simulink model "pll_stability_9bus"  (R2025b)
settings: Solver=ode23t  StartTime=0.0  StopTime=0.6  FixedStep=Ts  RelTol=1e-3  EnableMultiTasking=on
InitFcn:
  | proj_root = fileparts(get_param(bdroot, 'FileName'));
  | run(fullfile(proj_root, 'params.m'))
StopFcn:
  | run(fullfile(fileparts(get_param(bdroot, 'FileName')), 'scripts', 'export_sim_data.m'))
values from neighbouring files (symbols this model uses):
  C1 = 4.247098756978487e-05    (= 4.24709875698e-05)    [GridTiedInverterOptimalIData.m]    (also in params.m)
  den_notch_d = [1.0, -1.9198159829792367, 0.9417686752314415]    [params.m]
  Ki = 7075.557375636462 /4    (= 1768.88934391)    [GridTiedInverterOptimalIData.m]    (also in params.m)
  ki_pll = ki_pll * 0.2    (= 21164)    [params.m]
  Kp = 29.481489065151926 /4    (= 7.37037226629)    [GridTiedInverterOptimalIData.m]    (also in params.m)
  kp_pll = kp_pll * 0.2    (= 92)    [params.m]
  L1 = 0.03042088602562317    (= 0.0304208860256)    [GridTiedInverterOptimalIData.m]    (also in params.m)
  L2 = 0.0002889984172434201    (= 0.000288998417243)    [GridTiedInverterOptimalIData.m]    (also in params.m)
  num_notch_d = [0.9723401207349347, -1.9198159829792367, 0.9694285544965067]    [params.m]
  qsi = 0.707    [GridTiedInverterOptimalIData.m]    (also in params.m)
  Rd1 = 0.5734201923227409    (= 0.573420192323)    [GridTiedInverterOptimalIData.m]    (also in params.m)
  Rd2 = 0.0054474918270660385    (= 0.00544749182707)    [GridTiedInverterOptimalIData.m]    (also in params.m)
  Rd3 = 3.1228169353331086    (= 3.12281693533)    [GridTiedInverterOptimalIData.m]    (also in params.m)
  Ts = 5e-6    (= 5e-06)    [GridTiedInverterOptimalIData.m]    (also in params.m)
  Tsc = 2e-4    (= 0.0002)    [GridTiedInverterOptimalIData.m]    (also in params.m)
  Vcc = 90909.09090909091*1.5    (= 136363.636364)    [GridTiedInverterOptimalIData.m]    (also in params.m)
  wres = 9068.99682117109    (= 9068.99682117)    [GridTiedInverterOptimalIData.m]    (also in params.m)
libraries: nesl_utility x80, ee_lib x71, fl_lib x28, eeGeneralControl x9, eeTransforms x4, eeSmAC1C x3, eeSmPSS1A x3, simulink x3, eeSinusoidalMeasurement x1
(part 3 of 3)

== system pll_stability_9bus/Gen3@Bus3 PV 1.025 pu 85 MW/Governor and Prime Mover ==
  "Governor and Prime Mover " : Subsystem  mask(Governor and Prime Mover){droop_percentage=5, Tg=0.15, Tch=0.3, pu_torque0=0.668315, Ts=Ts}
      mask prompts: droop_percentage "Percentage droop, (%)"; Tg "Time constant of governor, Tg (s)"; Tch "Time constant of main inlet volumes and steam chest, Tch (s)"; pu_torque0 "Initial torque, (pu)"; Ts "Sample time"
      mask help:
      | Implements a synchronous machine governor and prime mover. The prime mover is a non-reheat steam turbine.
      |
      | The input to the block is a per-unit synchronous machine measurement vector.
      |
      | R and C are mechanical rotational ports.
  Mechanical Power : ee_lib/Electromechanical/Mechanical/Machine Mechanical Power  power_sign=-1  SRated=128 MW  FRated=60 Hz  nPolePairs=1  inputUnit=ee.enum.unit.pu  torque_factor=2  inertia_option=2  J=27548 kg*m^2  H=301/128 W*s/(A*V)  damper_option=2  D=39.0509 N*m*s/rad  pu_D=0  initialization_option=2  fMechanical0=60 Hz  fElectrical0=60 Hz
      settings: InternalSimscapePortConfiguration="{\"Bottom\":[],\"Left\":[{\"id\":\"Pm_pu\",\"label\":\"pu\",\"type\":\"input\"}],\"Right\":[{\"id\":\"R\",\"label\":\"R\",\"type\":\"foundation.mechanical.rotational.rotational\"},{\"id\":\"C\",\"label\":\"C\",\"type\":\"foundation.mechanical.rotational.rotational\"}],\"Top\":[]}"
  PS-Simulink Converter : nesl_utility/PS-Simulink Converter  PhysicalDomain=network_engine_domain  SubClassName=ps_output  LeftPortType=input  RightPortType=output  PseudoPeriodic=off  Frequencies=[]  VectorFormat=1-D array  Unit=1  AffineConversion=off
  Pref : Constant  Value=85/128
  Rotor velocity measurement : ee_lib/Electromechanical/Synchronous/Synchronous Machine Measurement  output_idx=4
      settings: InternalSimscapePortConfiguration="{\"Bottom\":[],\"Left\":[{\"id\":\"pu_input\",\"label\":\"pu\",\"type\":\"input\"}],\"Right\":[{\"id\":\"pu_output\",\"label\":\"o\",\"type\":\"output\"}],\"Top\":[]}"
  Simulink-PS Converter : nesl_utility/Simulink-PS Converter  PhysicalDomain=network_engine_domain  SubClassName=ps_input  LeftPortType=input  RightPortType=output  PseudoPeriodic=off  Frequencies=[]  NoiseDistribution=none  NoiseParameters=[]  Unit=1  AffineConversion=off  FilteringAndDerivatives=provide  SimscapeFilterOrder=1  InputFilterTimeConstant=0.001  UdotUserProvided=0
  Unit Delay : UnitDelay  InitialCondition=1  SampleTime=Ts  HasFrameUpgradeWarning=on
  wref : Constant
  R : PMIOPort  Side=Right
  C : PMIOPort  Port=2  Side=Right
  pu : PMIOPort  Port=3  Side=Left
  wires:
  PS-Simulink Converter/1 -> Unit Delay/1
  Unit Delay/1 -> "Governor and Prime Mover "/3(w)
  Pref/1 -> "Governor and Prime Mover "/2(Pref)
  "Governor and Prime Mover "/1(Tm) -> Simulink-PS Converter/1
  wref/1 -> "Governor and Prime Mover "/1(wref)
  connections:
  PS-Simulink Converter/LConn1 -- Rotor velocity measurement/RConn1
  Mechanical Power/RConn1 -- R/RConn1
  pu/RConn1 -- Rotor velocity measurement/LConn1
  Mechanical Power/RConn2 -- C/RConn1
  Mechanical Power/LConn1 -- Simulink-PS Converter/RConn1

== system pll_stability_9bus/UFV Model/Gate driver ==
  S : Inport
  Data Type Conversion : DataTypeConversion  OutDataTypeStr=double  SaturateOnIntegerOverflow=off  RndMeth=Floor
  Demux : Demux  Outputs=6
  Scope : Scope
      settings: ActiveDisplayYMinimum=-0.036991199119911888  ActiveDisplayYMaximum=1.0342409240924093  DataLoggingVariableName=ScopeData3
  Simulink-PS Converter{,1..5} (6 alike) : nesl_utility/Simulink-PS Converter  PhysicalDomain=network_engine_domain  SubClassName=ps_input  LeftPortType=input  RightPortType=output  PseudoPeriodic=off  Frequencies=[]  NoiseDistribution=none  NoiseParameters=[]  Unit=1  AffineConversion=off  FilteringAndDerivatives=provide  SimscapeFilterOrder=1  InputFilterTimeConstant=0.001  UdotUserProvided=0
  Six-Pulse Gate Multiplexer : ee_lib/Semiconductors & Converters/Converters/Six-Pulse Gate Multiplexer  port_option=ee.enum.controlport.ps
  G : PMIOPort  Side=Right
  wires:
  Demux/5 -> Simulink-PS Converter4/1
  Demux/3 -> Simulink-PS Converter2/1
  Data Type Conversion/1 -> Demux/1
  Demux/4 -> Simulink-PS Converter3/1
  Demux/6 -> Simulink-PS Converter5/1
  Demux/2 -> Simulink-PS Converter1/1
  Demux/1 -> Scope/1, Simulink-PS Converter/1
  S/1 -> Data Type Conversion/1
  connections:
  Simulink-PS Converter4/RConn1 -- Six-Pulse Gate Multiplexer/LConn5
  Simulink-PS Converter2/RConn1 -- Six-Pulse Gate Multiplexer/LConn3
  Simulink-PS Converter/RConn1 -- Six-Pulse Gate Multiplexer/LConn1
  Simulink-PS Converter5/RConn1 -- Six-Pulse Gate Multiplexer/LConn6
  Simulink-PS Converter1/RConn1 -- Six-Pulse Gate Multiplexer/LConn2
  Simulink-PS Converter3/RConn1 -- Six-Pulse Gate Multiplexer/LConn4
  Six-Pulse Gate Multiplexer/RConn1 -- G/RConn1

== system pll_stability_9bus/UFV Model/Measurement inverter ==
  Current and Voltage Sensor (Three-Phase) : ee_lib/Sensors & Transducers/Current and Voltage Sensor (Three-Phase)  vMeasurementType=2  outputUnit=1  SRated=100e6 V*A  VRated=18e3 V  I_specify=off  I_priority=None  I=[ 0 0 0 ] A  I_nominal_specify=off  I_nominal_value=1  I_nominal_unit=A  V_specify=off  V_priority=None  V=[ 0 0 0 ] V  V_nominal_specify=off  V_nominal_value=1  V_nominal_unit=V
      settings: InternalSimscapePortConfiguration="{\"Bottom\":[],\"Left\":[{\"id\":\"a1\",\"label\":\"a1\",\"type\":\"foundation.electrical.electrical\"},{\"id\":\"b1\",\"label\":\"b1\",\"type\":\"foundation.electrical.electrical\"},{\"id\":\"c1\",\"label\":\"c1\",\"type\":\"foundation.electrical.electrical\"}],\"Right\":[{\"id\":\"V_output\",\"label\":\"V\",\"type\":\"output\"},{\"id\":\"I_output\",\"label\":\"I\",\"type\":\"output\"},{\"id\":\"a2\",\"label\":\"a2\",\"type\":\"foundation.electrical.electrical\"},{\"id\":\"b2\",\"label\":\"b2\",\"type\":\"foundation.electrical.electrical\"},{\"id\":\"c2\",\"label\":\"c2\",\"type\":\"foundation.electrical.electrical\"}],\"Top\":[]}"
  PS-Simulink Converter : nesl_utility/PS-Simulink Converter  PhysicalDomain=network_engine_domain  SubClassName=ps_output  LeftPortType=input  RightPortType=output  PseudoPeriodic=off  Frequencies=[]  VectorFormat=1-D array  Unit=V  AffineConversion=off
  PS-Simulink Converter2 : nesl_utility/PS-Simulink Converter  PhysicalDomain=network_engine_domain  SubClassName=ps_output  LeftPortType=input  RightPortType=output  PseudoPeriodic=off  Frequencies=[]  VectorFormat=1-D array  Unit=1  AffineConversion=off
  PS-Simulink Converter3 : nesl_utility/PS-Simulink Converter  PhysicalDomain=network_engine_domain  SubClassName=ps_output  LeftPortType=input  RightPortType=output  PseudoPeriodic=off  Frequencies=[]  VectorFormat=1-D array  Unit=1  AffineConversion=off
  Voltage Sensor : fl_lib/Electrical/Electrical Sensors/Voltage Sensor
  a1 : PMIOPort  Side=Left
  b1 : PMIOPort  Port=2  Side=Left
  a2 : PMIOPort  Port=3  Side=Right
  b2 : PMIOPort  Port=4  Side=Right
  c1 : PMIOPort  Port=5  Side=Left
  c2 : PMIOPort  Port=6  Side=Right
  tag scope: Iabc_inverter=global, Vab_inverter=global, Vabc_inverter=global
  wires:
  PS-Simulink Converter3/1 -> [Iabc_inverter]
  PS-Simulink Converter/1 -> [Vab_inverter]
  PS-Simulink Converter2/1 -> [Vabc_inverter]
  connections:
  b2/RConn1 -- Voltage Sensor/RConn2 -- Current and Voltage Sensor (Three-Phase)/RConn4
  a2/RConn1 -- Voltage Sensor/LConn1 -- Current and Voltage Sensor (Three-Phase)/RConn3
  Current and Voltage Sensor (Three-Phase)/RConn5 -- c2/RConn1
  Current and Voltage Sensor (Three-Phase)/LConn2 -- b1/RConn1
  Current and Voltage Sensor (Three-Phase)/LConn3 -- c1/RConn1
  Current and Voltage Sensor (Three-Phase)/LConn1 -- a1/RConn1
  PS-Simulink Converter2/LConn1 -- Current and Voltage Sensor (Three-Phase)/RConn1
  Current and Voltage Sensor (Three-Phase)/RConn2 -- PS-Simulink Converter3/LConn1
  PS-Simulink Converter/LConn1 -- Voltage Sensor/RConn1

== system pll_stability_9bus/UFV Model/Measurement inverter1 ==
  Current and Voltage Sensor (Three-Phase) : ee_lib/Sensors & Transducers/Current and Voltage Sensor (Three-Phase)  vMeasurementType=2  outputUnit=ee.enum.unit.si  SRated=100e6 V*A  VRated=20e3 V  I_specify=off  I_priority=None  I=[ 0 0 0 ] A  I_nominal_specify=off  I_nominal_value=1  I_nominal_unit=A  V_specify=off  V_priority=None  V=[ 0 0 0 ] V  V_nominal_specify=off  V_nominal_value=1  V_nominal_unit=V
      settings: InternalSimscapePortConfiguration="{\"Bottom\":[],\"Left\":[{\"id\":\"a1\",\"label\":\"a1\",\"type\":\"foundation.electrical.electrical\"},{\"id\":\"b1\",\"label\":\"b1\",\"type\":\"foundation.electrical.electrical\"},{\"id\":\"c1\",\"label\":\"c1\",\"type\":\"foundation.electrical.electrical\"}],\"Right\":[{\"id\":\"V_output\",\"label\":\"V\",\"type\":\"output\"},{\"id\":\"I_output\",\"label\":\"I\",\"type\":\"output\"},{\"id\":\"a2\",\"label\":\"a2\",\"type\":\"foundation.electrical.electrical\"},{\"id\":\"b2\",\"label\":\"b2\",\"type\":\"foundation.electrical.electrical\"},{\"id\":\"c2\",\"label\":\"c2\",\"type\":\"foundation.electrical.electrical\"}],\"Top\":[]}"
  PS-Simulink Converter : nesl_utility/PS-Simulink Converter  PhysicalDomain=network_engine_domain  SubClassName=ps_output  LeftPortType=input  RightPortType=output  PseudoPeriodic=off  Frequencies=[]  VectorFormat=1-D array  Unit=V  AffineConversion=off
  PS-Simulink Converter2 : nesl_utility/PS-Simulink Converter  PhysicalDomain=network_engine_domain  SubClassName=ps_output  LeftPortType=input  RightPortType=output  PseudoPeriodic=off  Frequencies=[]  VectorFormat=1-D array  Unit=1  AffineConversion=off
  PS-Simulink Converter3 : nesl_utility/PS-Simulink Converter  PhysicalDomain=network_engine_domain  SubClassName=ps_output  LeftPortType=input  RightPortType=output  PseudoPeriodic=off  Frequencies=[]  VectorFormat=1-D array  Unit=1  AffineConversion=off
  Voltage Sensor : fl_lib/Electrical/Electrical Sensors/Voltage Sensor
  a1 : PMIOPort  Side=Left
  b1 : PMIOPort  Port=2  Side=Left
  a2 : PMIOPort  Port=3  Side=Right
  b2 : PMIOPort  Port=4  Side=Right
  c1 : PMIOPort  Port=5  Side=Left
  c2 : PMIOPort  Port=6  Side=Right
  tag scope: Iabc=global, Vab=global, Vabc=global
  wires:
  PS-Simulink Converter2/1 -> [Vabc]
  PS-Simulink Converter3/1 -> [Iabc]
  PS-Simulink Converter/1 -> [Vab]
  connections:
  b2/RConn1 -- Voltage Sensor/RConn2 -- Current and Voltage Sensor (Three-Phase)/RConn4
  a2/RConn1 -- Voltage Sensor/LConn1 -- Current and Voltage Sensor (Three-Phase)/RConn3
  Current and Voltage Sensor (Three-Phase)/RConn5 -- c2/RConn1
  Current and Voltage Sensor (Three-Phase)/LConn2 -- b1/RConn1
  Current and Voltage Sensor (Three-Phase)/LConn3 -- c1/RConn1
  Current and Voltage Sensor (Three-Phase)/LConn1 -- a1/RConn1
  PS-Simulink Converter2/LConn1 -- Current and Voltage Sensor (Three-Phase)/RConn1
  Current and Voltage Sensor (Three-Phase)/RConn2 -- PS-Simulink Converter3/LConn1
  PS-Simulink Converter/LConn1 -- Voltage Sensor/RConn1

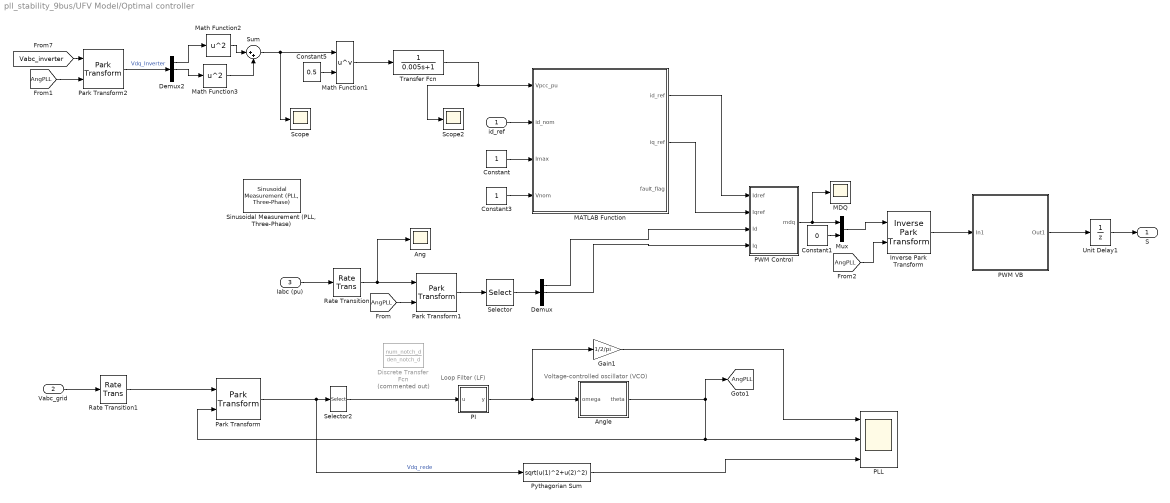
== system pll_stability_9bus/UFV Model/Optimal controller ==
  note: Loop Filter (LF)
  note: Voltage-controlled oscillator (VCO)
  id_ref : Inport
  Vabc_grid : Inport  Port=2
  Iabc (pu) : Inport  Port=3
  Ang : Scope
      settings: ActiveDisplayYMinimum=-3.3279661548723216  ActiveDisplayYMaximum=3.0621908527783015  DataLoggingVariableName=ScopeData7
  Angle : Subsystem
  Constant : Constant
  Constant1 : Constant  Value=0  SampleTime=Tsc
  Constant3 : Constant
  Constant5 : Constant  Value=0.5
  Demux : Demux  Outputs=3
  Demux2 : Demux  Outputs=3
  Discrete Transfer Fcn : DiscreteTransferFcn  Commented=on  Numerator=num_notch_d  Denominator=den_notch_d  InitialStates=[0 0]
  Gain1 : Gain  Gain=1/2/pi
  Inverse Park Transform : eeTransforms/Inverse Park Transform  AxisAlignment=Q-axis  PowerInvariant=off
  MATLAB Function : MATLAB Function  TreatAsAtomicUnit=on
  MDQ : Scope
      settings: ActiveDisplayYMinimum=-2.629038158512933  ActiveDisplayYMaximum=4.3781442766160286
  Math Function1 : Math  Operator=pow
  Math Function2 : Math  Operator=square
  Math Function3 : Math  Operator=square
  Mux : Mux  Inputs=2
  PI : Subsystem
  PLL : Scope  NumInputPorts=3
      settings: ActiveDisplayYMinimum=-0.78483497084376919  ActiveDisplayYMaximum=7.0635147375939251  DataLoggingVariableName=ScopeData27
  PWM Control : Subsystem
  PWM VB : Subsystem
  Park Transform : eeTransforms/Park Transform  AxisAlignment=Q-axis  PowerInvariant=off
  Park Transform1 : eeTransforms/Park Transform  AxisAlignment=Q-axis  PowerInvariant=off
  Park Transform2 : eeTransforms/Park Transform  AxisAlignment=Q-axis  PowerInvariant=off
  Pythagorian Sum : Fcn  Expr=sqrt(u(1)^2+u(2)^2)
  Rate Transition : RateTransition  OutPortSampleTime=Tsc
  Rate Transition1 : RateTransition  OutPortSampleTime=Tsc
  Scope : Scope
      settings: ActiveDisplayYMinimum=-1  ActiveDisplayYMaximum=1  DataLoggingVariableName=ScopeData22
  Scope2 : Scope
      settings: ActiveDisplayYMinimum=-1  ActiveDisplayYMaximum=1  DataLoggingVariableName=ScopeData23
  Selector : Selector  InputPortWidth=3  IndexOptions=Index vector (dialog)  Indices=[1 2 3]  OutputSizes=1
  Selector2 : Selector  InputPortWidth=3  IndexOptions=Index vector (dialog)  Indices=[2]  OutputSizes=1
  "Sinusoidal Measurement (PLL, Three-Phase)" : eeSinusoidalMeasurement/Sinusoidal Measurement (PLL, Three-Phase)  Kp_LF=460  Ki_LF=105820  F0=60  Theta0=0  Ts=Tsc
  Sum : Sum  Inputs=|++
  Transfer Fcn : TransferFcn  Denominator=[0.005 1]
  Unit Delay1 : UnitDelay  SampleTime=Ts  HasFrameUpgradeWarning=on
  S : Outport
  tag scope: AngPLL=global
  wires:
  Vabc_grid/1 -> Rate Transition1/1
  Iabc (pu)/1 -> Rate Transition/1
  Park Transform1/1 -> Selector/1
  Unit Delay1/1 -> S/1
  Rate Transition/1 -> Ang/1, Park Transform1/1
  Selector/1 -> Demux/1
  Demux/1 -> PWM Control/3(Id)
  Demux/2 -> PWM Control/4(Iq)
  PWM Control/1(mdq) -> MDQ/1, Mux/1
  Constant1/1 -> Mux/2
  Mux/1 -> Inverse Park Transform/1
  Inverse Park Transform/1 -> PWM VB/1(In1)
  PWM VB/1(Out1) -> Unit Delay1/1
  Constant/1 -> MATLAB Function/3(Imax)
  Constant3/1 -> MATLAB Function/4(Vnom)
  [Vabc_inverter] -> Park Transform2/1
  Constant5/1 -> Math Function1/2
  Math Function1/1 -> Transfer Fcn/1
  Park Transform2/1 -> Demux2/1  "Vdq_Inverter"
  Demux2/1 -> Math Function2/1
  Demux2/2 -> Math Function3/1
  Math Function2/1 -> Sum/1
  Math Function3/1 -> Sum/2
  Sum/1 -> Scope/1, Math Function1/1
  MATLAB Function/2(iq_ref) -> PWM Control/2(Iqref)
  id_ref/1 -> MATLAB Function/2(id_nom)
  MATLAB Function/1(id_ref) -> PWM Control/1(Idref)
  Transfer Fcn/1 -> MATLAB Function/1(Vpcc_pu), Scope2/1
  Gain1/1 -> PLL/1
  Park Transform/1 -> Selector2/1, Pythagorian Sum/1  "Vdq_rede"
  Angle/1(theta) -> [AngPLL], PLL/2, Park Transform/2
  PI/1(y) -> Angle/1(omega), Gain1/1
  Pythagorian Sum/1 -> PLL/3
  Rate Transition1/1 -> Park Transform/1
  Selector2/1 -> PI/1(u)
  [AngPLL] -> Park Transform1/2
  [AngPLL] -> Park Transform2/2
  [AngPLL] -> Inverse Park Transform/2

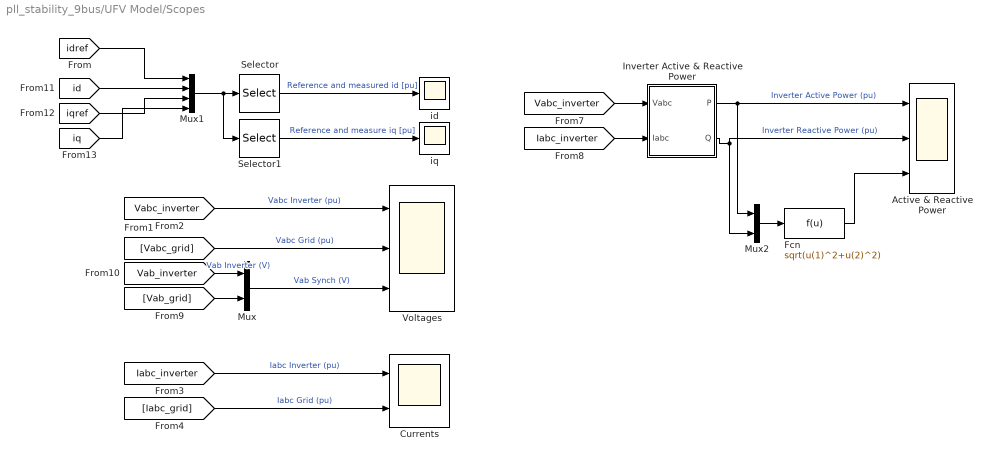
== system pll_stability_9bus/UFV Model/Scopes ==
  Active & Reactive Power : Scope  NumInputPorts=3
      settings: ActiveDisplayYMinimum=-1.7507657355303796  ActiveDisplayYMaximum=1.8726008267641796  DataLoggingDecimation=10
  Currents : Scope  NumInputPorts=2
      settings: ActiveDisplayYMinimum=-2.3032474961806439  ActiveDisplayYMaximum=2.7208093208856536  DataLoggingVariableName=ScopeData2
  Fcn : Fcn  Expr=sqrt(u(1)^2+u(2)^2)
  "Inverter Active & Reactive Power " : Subsystem
  Mux : Mux  Inputs=2
  Mux1 : Mux
  Mux2 : Mux  Inputs=2
  Selector : Selector  InputPortWidth=4  IndexOptions=Index vector (dialog)  Indices=[1 2]  OutputSizes=1
  Selector1 : Selector  InputPortWidth=4  IndexOptions=Index vector (dialog)  Indices=[3 4]  OutputSizes=1
  Voltages : Scope  NumInputPorts=3
      settings: ActiveDisplayYMinimum=-1.639643273335825  ActiveDisplayYMaximum=1.519858388794153  DataLoggingVariableName=ScopeData6
  id : Scope
      settings: ActiveDisplayYMinimum=-1.3315143959536515  ActiveDisplayYMaximum=2.0514500627668606
  iq : Scope
      settings: ActiveDisplayYMinimum=-2.6547417522691337  ActiveDisplayYMaximum=1.5619388517626811  DataLoggingVariableName=ScopeData2
  wires:
  [Vab_grid] -> Mux/2
  [Iabc_inverter] -> Currents/1  "Iabc Inverter (pu)"
  [Iabc_grid] -> Currents/2  "Iabc Grid (pu)"
  [Vabc_inverter] -> Voltages/1  "Vabc Inverter (pu)"
  [Vabc_inverter] -> "Inverter Active & Reactive Power "/1(Vabc)
  [Iabc_inverter] -> "Inverter Active & Reactive Power "/2(Iabc)
  "Inverter Active & Reactive Power "/1(P) -> Mux2/1, Active & Reactive Power/1  "Inverter Active Power (pu)"
  Mux/1 -> Voltages/3  "Vab Synch (V)"
  [Vab_inverter] -> Mux/1  "Vab Inverter (V)"
  "Inverter Active & Reactive Power "/2(Q) -> Mux2/2, Active & Reactive Power/2  "Inverter Reactive Power (pu)"
  [Vabc_grid] -> Voltages/2  "Vabc Grid (pu)"
  Mux1/1 -> Selector1/1, Selector/1
  Selector1/1 -> iq/1  "Reference and measure iq [pu]"
  [idref] -> Mux1/1
  Selector/1 -> id/1  "Reference and measured id [pu]"
  [id] -> Mux1/2
  [iqref] -> Mux1/3
  [iq] -> Mux1/4
  Mux2/1 -> Fcn/1
  Fcn/1 -> Active & Reactive Power/3

== system pll_stability_9bus/Gen1@Bus1 Swing/Governor and Prime Mover/Governor and Prime Mover  ==
  wref : Inport
  Pref : Inport  Port=2
  w : Inport  Port=3
  Governor : Subsystem
  Non-reheat turbine : Subsystem
  Tm : Outport  VectorParamsAs1DForOutWhenUnconnected=off
  wires:
  w/1 -> Governor/3(w)
  Pref/1 -> Governor/2(Pref)
  wref/1 -> Governor/1(wref)
  Non-reheat turbine/1(torque) -> Tm/1
  Governor/1(delta_y) -> Non-reheat turbine/1(delta_y)

== system pll_stability_9bus/Gen2@Bus2 PV 1.025 pu 163 MW/Governor and Prime Mover/Governor and Prime Mover  ==
  wref : Inport
  Pref : Inport  Port=2
  w : Inport  Port=3
  Governor : Subsystem
  Non-reheat turbine : Subsystem
  Tm : Outport  VectorParamsAs1DForOutWhenUnconnected=off
  wires:
  Governor/1(delta_y) -> Non-reheat turbine/1(delta_y)
  Non-reheat turbine/1(torque) -> Tm/1
  wref/1 -> Governor/1(wref)
  Pref/1 -> Governor/2(Pref)
  w/1 -> Governor/3(w)

== system pll_stability_9bus/Gen3@Bus3 PV 1.025 pu 85 MW/Governor and Prime Mover/Governor and Prime Mover  ==
  wref : Inport
  Pref : Inport  Port=2
  w : Inport  Port=3
  Governor : Subsystem
  Non-reheat turbine : Subsystem
  Tm : Outport  VectorParamsAs1DForOutWhenUnconnected=off
  wires:
  w/1 -> Governor/3(w)
  Pref/1 -> Governor/2(Pref)
  wref/1 -> Governor/1(wref)
  Non-reheat turbine/1(torque) -> Tm/1
  Governor/1(delta_y) -> Non-reheat turbine/1(delta_y)

== system pll_stability_9bus/UFV Model/Optimal controller/Angle ==
  omega : Inport
  Integrator with Wrapped State (Discrete or Continuous) : eeGeneralControl/Integrator with Wrapped State (Discrete or Continuous)  LabelModeActiveChoice=Discrete  WrappedStateUpperValue=2*pi  WrappedStateLowerValue=0  x0=0  Ts=Tsc
  theta : Outport  VectorParamsAs1DForOutWhenUnconnected=off
  wires:
  Integrator with Wrapped State (Discrete or Continuous)/1 -> theta/1
  omega/1 -> Integrator with Wrapped State (Discrete or Continuous)/1

== system pll_stability_9bus/UFV Model/Optimal controller/PI ==
  u : Inport
  Constant : Constant  Value=2*pi*60  SampleTime=Ts
  Constant1 : Constant  Value=0  SampleTime=Ts
  Data Type Conversion Inherited : simulink/Signal Attributes/Data Type Conversion Inherited  ConvertRealWorld=Real World Value  DoSatur=off
  Gain : Gain  Gain=kp_pll
  Gain1 : Gain  Gain=ki_pll
  Integrator (Discrete or Continuous) : eeGeneralControl/Integrator (Discrete or Continuous)  LabelModeActiveChoice=Discrete  IntegratorMethod=Integration: Forward Euler  ExternalReset=level  LimitType=Anti-windup  B=inf  A=-inf  Ts=Tsc
  Sum : Sum  Inputs=|++
  y : Outport  VectorParamsAs1DForOutWhenUnconnected=off
  wires:
  Constant/1 -> Data Type Conversion Inherited/2
  Data Type Conversion Inherited/1 -> Integrator (Discrete or Continuous)/3
  Gain1/1 -> Integrator (Discrete or Continuous)/1
  u/1 -> Gain1/1, Data Type Conversion Inherited/1, Gain/1
  Gain/1 -> Sum/1
  Integrator (Discrete or Continuous)/1 -> Sum/2
  Sum/1 -> y/1
  Constant1/1 -> Integrator (Discrete or Continuous)/2

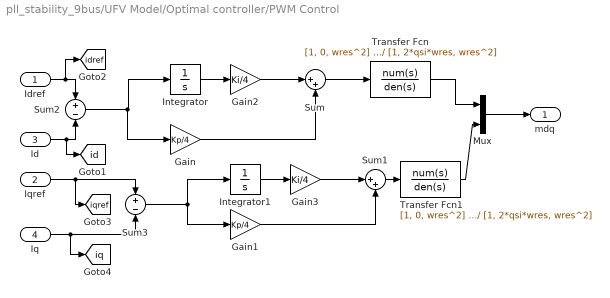
== system pll_stability_9bus/UFV Model/Optimal controller/PWM Control ==
  Idref : Inport
  Iqref : Inport  Port=2
  Id : Inport  Port=3
  Iq : Inport  Port=4
  Gain : Gain  Gain=Kp/4
  Gain1 : Gain  Gain=Kp/4
  Gain2 : Gain  Gain=Ki/4
  Gain3 : Gain  Gain=Ki/4
  Integrator : Integrator  LimitOutput=on  UpperSaturationLimit=2  LowerSaturationLimit=-2
  Integrator1 : Integrator  LimitOutput=on  UpperSaturationLimit=2  LowerSaturationLimit=-2
  Mux : Mux  Inputs=2
  Sum : Sum  Inputs=|++
  Sum1 : Sum  Inputs=|++
  Sum2 : Sum  Inputs=+-
  Sum3 : Sum  Inputs=+-
  Transfer Fcn : TransferFcn  Numerator=[1, 0, wres^2]  Denominator=[1, 2*qsi*wres, wres^2]
  Transfer Fcn1 : TransferFcn  Numerator=[1, 0, wres^2]  Denominator=[1, 2*qsi*wres, wres^2]
  mdq : Outport
  tag scope: id=global, idref=global, iq=global, iqref=global
  wires:
  Gain/1 -> Sum/2
  Gain1/1 -> Sum1/2
  Mux/1 -> mdq/1
  Sum3/1 -> Gain1/1, Integrator1/1
  Sum/1 -> Transfer Fcn/1
  Gain2/1 -> Sum/1
  Sum2/1 -> Gain/1, Integrator/1
  Transfer Fcn1/1 -> Mux/2
  Gain3/1 -> Sum1/1
  Integrator1/1 -> Gain3/1
  Integrator/1 -> Gain2/1
  Transfer Fcn/1 -> Mux/1
  Iq/1 -> [iq], Sum3/2
  Sum1/1 -> Transfer Fcn1/1
  Idref/1 -> [idref], Sum2/1
  Id/1 -> [id], Sum2/2
  Iqref/1 -> [iqref], Sum3/1

== system pll_stability_9bus/UFV Model/Optimal controller/PWM VB ==
  In1 : Inport
  Comparador PWM : Scope  NumInputPorts=2
      settings: ActiveDisplayYMinimum=-4.9312706623685774  ActiveDisplayYMaximum=4.5345736038914586  DataLoggingVariableName=ScopeData4
  Demux1 : Demux  Outputs=3
  Logical Operator3 : Logic  Operator=NOT  AllPortsSameDT=off  OutDataTypeStr=boolean
  Mux1 : Mux  Inputs=3
  Mux2 : Mux  Inputs=2
  Relational Operator : RelationalOperator  OutDataTypeStr=boolean  RndMeth=Simplest  InputSameDT=off
  Relational Operator1 : RelationalOperator  OutDataTypeStr=boolean  RndMeth=Simplest  InputSameDT=off
  Relational Operator2 : RelationalOperator  OutDataTypeStr=boolean  RndMeth=Simplest  InputSameDT=off
  Repeating Sequence : simulink/Sources/Repeating Sequence  rep_seq_t=[0, 0.00005, 0.0001, 0.00015, 0.0002]  rep_seq_y=[0, 1, 0, -1, 0]
  Selector1 : Selector  InputPortWidth=6  IndexOptions=Index vector (dialog)  Indices=[1 4 2 5 3 6]  OutputSizes=1
  Out1 : Outport
  wires:
  Demux1/3 -> Relational Operator2/1
  Repeating Sequence/1 -> Relational Operator2/2, Relational Operator1/2, Relational Operator/2, Comparador PWM/1
  Mux2/1 -> Selector1/1
  Relational Operator2/1 -> Mux1/3
  Demux1/1 -> Relational Operator/1, Comparador PWM/2
  Mux1/1 -> Mux2/1, Logical Operator3/1
  Demux1/2 -> Relational Operator1/1
  Logical Operator3/1 -> Mux2/2
  Relational Operator1/1 -> Mux1/2
  Relational Operator/1 -> Mux1/1
  Selector1/1 -> Out1/1
  In1/1 -> Demux1/1

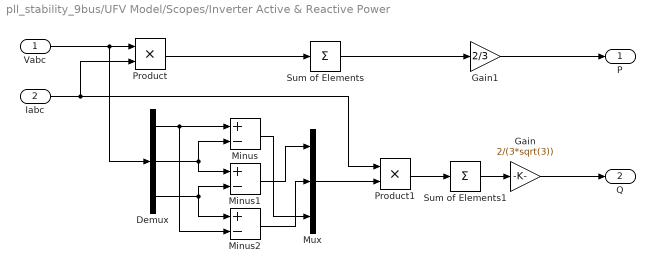
== system pll_stability_9bus/UFV Model/Scopes/Inverter Active & Reactive Power  ==
  Vabc : Inport
  Iabc : Inport  Port=2
  Demux : Demux  Outputs=3
  Gain : Gain  Gain=2/(3*sqrt(3))
  Gain1 : Gain  Gain=2/3
  Minus : Sum  Inputs=+-
  Minus1 : Sum  Inputs=+-
  Minus2 : Sum  Inputs=+-
  Mux : Mux  Inputs=3
  Product : Product
  Product1 : Product
  Sum of Elements : Sum  Inputs=+
  Sum of Elements1 : Sum  Inputs=+
  P : Outport  VectorParamsAs1DForOutWhenUnconnected=off
  Q : Outport  Port=2  VectorParamsAs1DForOutWhenUnconnected=off
  wires:
  Minus/1 -> Mux/3
  Minus2/1 -> Mux/2
  Minus1/1 -> Mux/1
  Gain/1 -> Q/1
  Sum of Elements1/1 -> Gain/1
  Product1/1 -> Sum of Elements1/1
  Mux/1 -> Product1/2
  Demux/3 -> Minus1/2, Minus2/1
  Demux/2 -> Minus/2, Minus1/1
  Demux/1 -> Minus/1, Minus2/2
  Sum of Elements/1 -> Gain1/1
  Product/1 -> Sum of Elements/1
  Iabc/1 -> Product/2, Product1/1
  Vabc/1 -> Product/1, Demux/1
  Gain1/1 -> P/1

== system pll_stability_9bus/Gen1@Bus1 Swing/Governor and Prime Mover/Governor and Prime Mover /Governor ==
  wref : Inport
  Pref : Inport  Port=2
  w : Inport  Port=3
  1/Tg : Gain  Gain=1/Tg
  1/droop : Gain  Gain=1/(droop_percentage/100)
  Constant : Constant  Value=pu_torque0
  Constant1 : Constant  Value=0
  Delta load setpoint : Sum  Inputs=+-|
  Delta speed : Sum  Inputs=-+|
  Integrator (Discrete or Continuous) : eeGeneralControl/Integrator (Discrete or Continuous)  LabelModeActiveChoice=Discrete  IntegratorMethod=Integration: Forward Euler  ExternalReset=level  LimitType=Anti-windup  B=inf  A=-inf  Ts=Ts
  Subtract : Sum  Inputs=|+-
  delta_y : Outport  VectorParamsAs1DForOutWhenUnconnected=off
  wires:
  Constant1/1 -> Integrator (Discrete or Continuous)/2
  Constant/1 -> Integrator (Discrete or Continuous)/3
  Pref/1 -> Delta load setpoint/1
  wref/1 -> Delta speed/1
  Integrator (Discrete or Continuous)/1 -> Subtract/2, delta_y/1
  1/Tg/1 -> Integrator (Discrete or Continuous)/1
  Subtract/1 -> 1/Tg/1
  Delta load setpoint/1 -> Subtract/1
  1/droop/1 -> Delta load setpoint/2
  w/1 -> Delta speed/2
  Delta speed/1 -> 1/droop/1

== system pll_stability_9bus/Gen1@Bus1 Swing/Governor and Prime Mover/Governor and Prime Mover /Non-reheat turbine ==
  delta_y : Inport
  1/Tch : Gain  Gain=1/Tch
  Constant : Constant  Value=pu_torque0
  Constant1 : Constant  Value=0
  Integrator (Discrete or Continuous) : eeGeneralControl/Integrator (Discrete or Continuous)  LabelModeActiveChoice=Discrete  IntegratorMethod=Integration: Forward Euler  ExternalReset=level  LimitType=Anti-windup  B=inf  A=-inf  Ts=Ts
  Sum : Sum  Inputs=|+-
  torque : Outport  VectorParamsAs1DForOutWhenUnconnected=off
  wires:
  Constant/1 -> Integrator (Discrete or Continuous)/3
  Constant1/1 -> Integrator (Discrete or Continuous)/2
  Integrator (Discrete or Continuous)/1 -> torque/1, Sum/2
  1/Tch/1 -> Integrator (Discrete or Continuous)/1
  Sum/1 -> 1/Tch/1
  delta_y/1 -> Sum/1

== system pll_stability_9bus/Gen2@Bus2 PV 1.025 pu 163 MW/Governor and Prime Mover/Governor and Prime Mover /Governor ==
  wref : Inport
  Pref : Inport  Port=2
  w : Inport  Port=3
  1/Tg : Gain  Gain=1/Tg
  1/droop : Gain  Gain=1/(droop_percentage/100)
  Constant : Constant  Value=pu_torque0
  Constant1 : Constant  Value=0
  Delta load setpoint : Sum  Inputs=+-|
  Delta speed : Sum  Inputs=-+|
  Integrator (Discrete or Continuous) : eeGeneralControl/Integrator (Discrete or Continuous)  LabelModeActiveChoice=Discrete  IntegratorMethod=Integration: Forward Euler  ExternalReset=level  LimitType=Anti-windup  B=inf  A=-inf  Ts=Ts
  Subtract : Sum  Inputs=|+-
  delta_y : Outport  VectorParamsAs1DForOutWhenUnconnected=off
  wires:
  Delta speed/1 -> 1/droop/1
  w/1 -> Delta speed/2
  1/droop/1 -> Delta load setpoint/2
  Delta load setpoint/1 -> Subtract/1
  Subtract/1 -> 1/Tg/1
  1/Tg/1 -> Integrator (Discrete or Continuous)/1
  Integrator (Discrete or Continuous)/1 -> delta_y/1, Subtract/2
  wref/1 -> Delta speed/1
  Pref/1 -> Delta load setpoint/1
  Constant/1 -> Integrator (Discrete or Continuous)/3
  Constant1/1 -> Integrator (Discrete or Continuous)/2

== system pll_stability_9bus/Gen2@Bus2 PV 1.025 pu 163 MW/Governor and Prime Mover/Governor and Prime Mover /Non-reheat turbine ==
  delta_y : Inport
  1/Tch : Gain  Gain=1/Tch
  Constant : Constant  Value=pu_torque0
  Constant1 : Constant  Value=0
  Integrator (Discrete or Continuous) : eeGeneralControl/Integrator (Discrete or Continuous)  LabelModeActiveChoice=Discrete  IntegratorMethod=Integration: Forward Euler  ExternalReset=level  LimitType=Anti-windup  B=inf  A=-inf  Ts=Ts
  Sum : Sum  Inputs=|+-
  torque : Outport  VectorParamsAs1DForOutWhenUnconnected=off
  wires:
  delta_y/1 -> Sum/1
  Sum/1 -> 1/Tch/1
  1/Tch/1 -> Integrator (Discrete or Continuous)/1
  Integrator (Discrete or Continuous)/1 -> Sum/2, torque/1
  Constant1/1 -> Integrator (Discrete or Continuous)/2
  Constant/1 -> Integrator (Discrete or Continuous)/3

== system pll_stability_9bus/Gen3@Bus3 PV 1.025 pu 85 MW/Governor and Prime Mover/Governor and Prime Mover /Governor ==
  wref : Inport
  Pref : Inport  Port=2
  w : Inport  Port=3
  1/Tg : Gain  Gain=1/Tg
  1/droop : Gain  Gain=1/(droop_percentage/100)
  Constant : Constant  Value=pu_torque0
  Constant1 : Constant  Value=0
  Delta load setpoint : Sum  Inputs=+-|
  Delta speed : Sum  Inputs=-+|
  Integrator (Discrete or Continuous) : eeGeneralControl/Integrator (Discrete or Continuous)  LabelModeActiveChoice=Discrete  IntegratorMethod=Integration: Forward Euler  ExternalReset=level  LimitType=Anti-windup  B=inf  A=-inf  Ts=Ts
  Subtract : Sum  Inputs=|+-
  delta_y : Outport  VectorParamsAs1DForOutWhenUnconnected=off
  wires:
  Constant1/1 -> Integrator (Discrete or Continuous)/2
  Constant/1 -> Integrator (Discrete or Continuous)/3
  Pref/1 -> Delta load setpoint/1
  wref/1 -> Delta speed/1
  Integrator (Discrete or Continuous)/1 -> Subtract/2, delta_y/1
  1/Tg/1 -> Integrator (Discrete or Continuous)/1
  Subtract/1 -> 1/Tg/1
  Delta load setpoint/1 -> Subtract/1
  1/droop/1 -> Delta load setpoint/2
  w/1 -> Delta speed/2
  Delta speed/1 -> 1/droop/1

== system pll_stability_9bus/Gen3@Bus3 PV 1.025 pu 85 MW/Governor and Prime Mover/Governor and Prime Mover /Non-reheat turbine ==
  delta_y : Inport
  1/Tch : Gain  Gain=1/Tch
  Constant : Constant  Value=pu_torque0
  Constant1 : Constant  Value=0
  Integrator (Discrete or Continuous) : eeGeneralControl/Integrator (Discrete or Continuous)  LabelModeActiveChoice=Discrete  IntegratorMethod=Integration: Forward Euler  ExternalReset=level  LimitType=Anti-windup  B=inf  A=-inf  Ts=Ts
  Sum : Sum  Inputs=|+-
  torque : Outport  VectorParamsAs1DForOutWhenUnconnected=off
  wires:
  Constant/1 -> Integrator (Discrete or Continuous)/3
  Constant1/1 -> Integrator (Discrete or Continuous)/2
  Integrator (Discrete or Continuous)/1 -> torque/1, Sum/2
  1/Tch/1 -> Integrator (Discrete or Continuous)/1
  Sum/1 -> 1/Tch/1
  delta_y/1 -> Sum/1

== matlab function pll_stability_9bus/UFV Model/Optimal controller/MATLAB Function ==
  data: Vpcc_pu input; id_ref output; id_nom input; Imax input; Vnom input; iq_ref output; fault_flag output
function [id_ref, iq_ref, fault_flag] = ONS_2_11(Vpcc_pu, id_nom, Imax, Vnom)

    V_mag = Vpcc_pu;

    % Ganhos definidos pelos pontos
    k_low = (0 -(- 1)) / (0.85 - 0.5);   % ≈ 2.857
    k_high = (1 - 0) / (1.2 - 1.1);  % = 10
    
    % Interceptos
    b_low = -k_low * 0.85;   % ≈ -2.4286
    b_high = -k_high * 1.1;  % = -11

    if V_mag < 0.85
        % 🔻 SUBTENSÃO
        fault_flag = 1;
        
        iq_ref_raw = k_low * V_mag + b_low;
        iq_ref = max(min(iq_ref_raw, Imax), -Imax);

        id_max_available = sqrt(max(Imax^2 - iq_ref^2, 0));
        id_ref = min(id_nom, id_max_available);

    elseif V_mag > 1.1
        % 🔺 SOBRETENSÃO
        fault_flag = 1;
        
        iq_ref_raw = k_high * V_mag + b_high;
        iq_ref = max(min(iq_ref_raw, Imax), -Imax);

        id_max_available = sqrt(max(Imax^2 - iq_ref^2, 0));
        id_ref = min(id_nom, id_max_available);

    else
        % ✅ REGIÃO NORMAL
        fault_flag = 0;
        id_ref = id_nom;
        iq_ref = 0;
    end
end
